simulink model "Robot_3gdl_PRR_Forward"  (R2014a)
settings: Solver=ode3  StartTime=0.0  StopTime=9.99  FixedStep=0.03  RelTol=1e-3
values from neighbouring files (symbols this model uses):
  RobotPRR = SerialLink(L,'name','PRR')    [IniciaParametrosPRR.m]
libraries: roblocks x3
settings Model: Creator=corkep  LastModifiedBy=fertape
settings DataIOCC: SignalLoggingSaveFormat=ModelDataLogs
settings OptimizationCC: ExpressionDepthLimit=2147483647
settings DebuggingCC: UnderspecifiedInitializationDetection=Classic  FcnCallInpInsideContextMsg=UseLocalSettings  StateNameClashWarn=warning
settings GRTTargetCC: CombineOutputUpdateFcns=off  GRTInterface=on

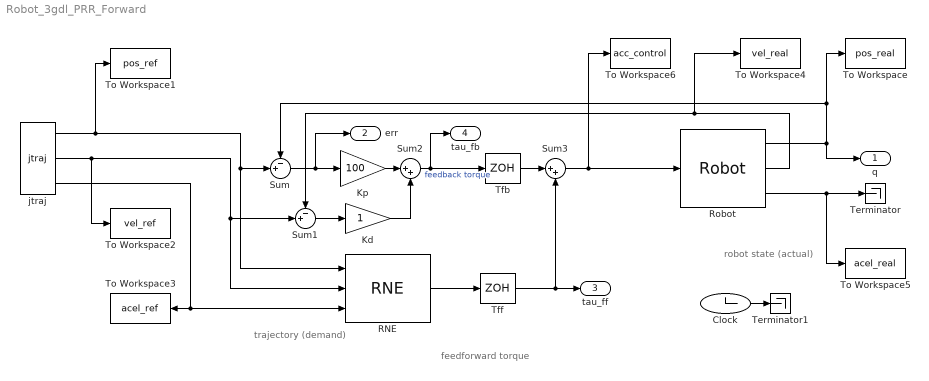
== system Robot_3gdl_PRR_Forward ==
  note: trajectory
      | (demand)
  note: robot state
      | (actual)
  note: feedforward torque
  Clock : Clock
  Kd : Gain  SaturateOnIntegerOverflow=on  OutDataTypeStr=Inherit: Same as input  ParamDataTypeStr=Inherit: Same as input
  Kp : Gain  Gain=100  SaturateOnIntegerOverflow=on  OutDataTypeStr=Inherit: Same as input  ParamDataTypeStr=Inherit: Same as input
  RNE : roblocks/Dynamics/RNE  robot=RobotPRR.nofriction()  grav=gravedad
  Robot : roblocks/Dynamics/Robot  robot=RobotPRR  q0=Qini
  Sum : Sum  Inputs=-+|  SaturateOnIntegerOverflow=on  InputSameDT=on  OutDataTypeStr=Inherit: Same as first input
  Sum1 : Sum  Inputs=-+|  SaturateOnIntegerOverflow=on  InputSameDT=on  OutDataTypeStr=Inherit: Same as first input
  Sum2 : Sum  Inputs=|++  SaturateOnIntegerOverflow=on  InputSameDT=on  OutDataTypeStr=Inherit: Same as first input
  Sum3 : Sum  Inputs=|++  SaturateOnIntegerOverflow=on  InputSameDT=on  OutDataTypeStr=Inherit: Same as first input
  Terminator : Terminator
  Terminator1 : Terminator
  Tfb : ZeroOrderHold  SampleTime=0.03
  Tff : ZeroOrderHold  SampleTime=0.03
  To Workspace : ToWorkspace  VariableName=pos_real  SaveFormat=Structure With Time  SampleTime=-1
  To Workspace1 : ToWorkspace  VariableName=pos_ref  SaveFormat=Structure With Time  SampleTime=-1
  To Workspace2 : ToWorkspace  VariableName=vel_ref  SaveFormat=Structure With Time  SampleTime=-1
  To Workspace3 : ToWorkspace  VariableName=acel_ref  SaveFormat=Structure With Time  SampleTime=-1
  To Workspace4 : ToWorkspace  VariableName=vel_real  SaveFormat=Structure With Time  SampleTime=-1
  To Workspace5 : ToWorkspace  VariableName=acel_real  SaveFormat=Structure With Time  SampleTime=-1
  To Workspace6 : ToWorkspace  VariableName=acc_control  SaveFormat=Structure With Time  SampleTime=-1
  jtraj : roblocks/Trajectory/jtraj  q0=Qini  qf=Qfin  tmax=10  ts=0.03
  q : Outport
  err : Outport  Port=2
  tau_ff : Outport  Port=3
  tau_fb : Outport  Port=4
  wires:
  Kd/1 -> Sum2/2
  Sum/1 -> Kp/1, err/1
  Kp/1 -> Sum2/1
  Sum1/1 -> Kd/1
  Sum2/1 -> Tfb/1, tau_fb/1  "feedback torque"
  Sum3/1 -> To Workspace6/1, Robot/1
  Robot/1 -> q/1, To Workspace/1, Sum/1
  Robot/2 -> To Workspace4/1, Sum1/1
  jtraj/1 -> RNE/1, Sum/2, To Workspace1/1
  jtraj/2 -> Sum1/2, RNE/2, To Workspace2/1
  jtraj/3 -> To Workspace3/1, RNE/3
  Robot/3 -> To Workspace5/1, Terminator/1
  Tff/1 -> Sum3/2, tau_ff/1
  Tfb/1 -> Sum3/1
  RNE/1 -> Tff/1
  Clock/1 -> Terminator1/1
